simulink model "Neww"  (R2016a)
settings: Solver=VariableStepAuto  StartTime=0.0  StopTime=4  RelTol=1e-3
libraries: fl_lib x10, elec_lib x5, simrfV2util1 x1, nesl_utility x1
settings Model: Creator=syf  LastModifiedBy=syf
settings DebuggingCC: AlgebraicLoopMsg=none  ArtificialAlgebraicLoopMsg=none

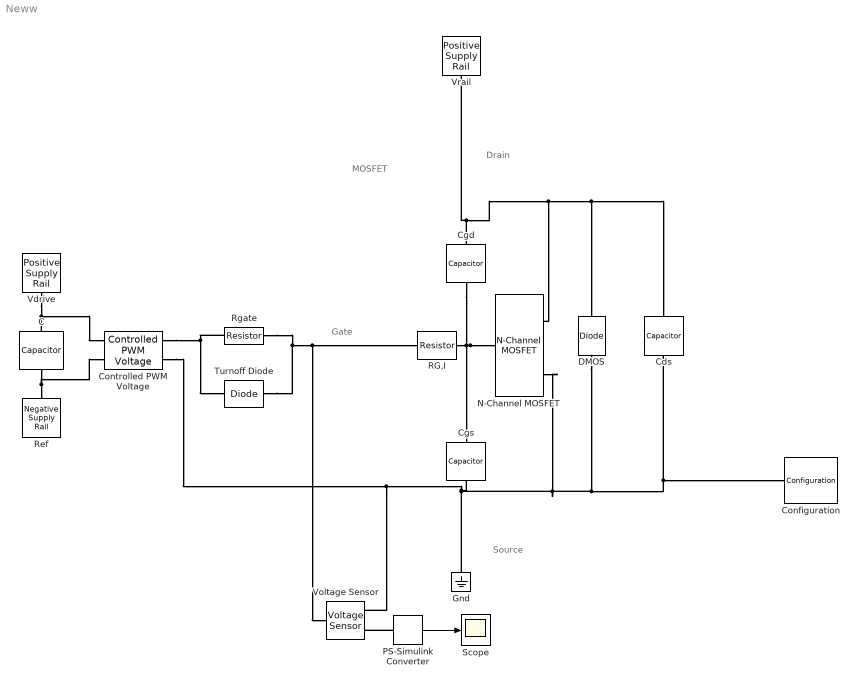
== system Neww ==
  note: Source
  note: Drain
  note: Gate
  note: MOSFET
  C : fl_lib/Electrical/Electrical Elements/Capacitor  c=0.4e-9 F  r=1e-6 Ohm  g=0 1/Ohm  i_specify=off  i_priority=None  i=0 A  v_specify=off  v_priority=None  v=0 V  vc_specify=off  vc_priority=High  vc=0 V
  Cds : fl_lib/Electrical/Electrical Elements/Capacitor  c=0.4e-9 F  r=1e-6 Ohm  g=0 1/Ohm  i_specify=off  i_priority=None  i=0 A  v_specify=off  v_priority=None  v=0 V  vc_specify=off  vc_priority=High  vc=0 V
  Cgd : fl_lib/Electrical/Electrical Elements/Capacitor  c=0.4e-9 F  r=1e-6 Ohm  g=0 1/Ohm  i_specify=off  i_priority=None  i=0 A  v_specify=off  v_priority=None  v=0 V  vc_specify=off  vc_priority=High  vc=0 V
  Cgs : fl_lib/Electrical/Electrical Elements/Capacitor  c=0.4e-9 F  r=1e-6 Ohm  g=0 1/Ohm  i_specify=off  i_priority=None  i=0 A  v_specify=off  v_priority=None  v=0 V  vc_specify=off  vc_priority=High  vc=0 V
  Configuration : simrfV2util1/Configuration  AutoFreq=on  Tones=[] Hz  Harmonics=[]  NormalizeCarrierPower=on  SolverType=Auto  StepSize=1e-6 s  AddNoise=on  Temperature=290.0 K  SolverDelFlag=0
  Controlled PWM Voltage : elec_lib/Actuators & Drivers/Drivers/Controlled PWM Voltage  F=1000 Hz  TD=0 s  pulse_width_offset=0 s  Vmin=0 V  Vmax=5 V  Vm=5 V  pwm_or_av=1  event_type=1  sample_time=1e-6 s
  DMOS : fl_lib/Electrical/Electrical Elements/Diode  Vf=0.6 V  Ron=0.1 Ohm  Goff=1e-8 1/Ohm  i_specify=off  i_priority=None  i=0 A  v_specify=off  v_priority=None  v=0 V
  Gnd : fl_lib/Electrical/Electrical Elements/Electrical Reference
  N-Channel MOSFET : elec_lib/Semiconductor Devices/N-Channel MOSFET  parameterization=1  prmDatasheet=1  prmEquCoeff=1  Beta=5 A/V^2  Rds=0.025 Ohm  Id=6 A  Vgs=10 V  Vth=1.3 V  lam=0 1/V  Tmeas=25 degC  RS=1e-4 Ohm  RD=0.01 Ohm  C_param=1  C_GS=270 pF  C_GD=80 pF  C_DS=0 pF  C_iss=350 pF  C_rss=80 pF  C_oss=0 pF  C_GS_vec=[ 270 300 290 280 295 255 ] pF  C_GD_vec=[ 450 400 300 190 95 55 ] pF  C_DS_vec=[ 450 410 390 230 175 115 ] pF  C_iss_vec=[ 720 700 590 470 390 310 ] pF  C_rss_vec=[ 450 400 300 190 95 55 ] pF  C_oss_vec=[ 900 810 690 420 270 170 ] pF  C_Vds_vec=[ 0.1 0.3 1 3 10 30 ] V  charge_linearity_param=1  C_OX=200 pF  V_C_OX=-0.5 V  dVth_dT=-6 mV/K  Rds_T2=0.037 Ohm  Tmeas2=125 degC  BEXDatasheet=-1.5  BEXEquCoeff=-1.5  TdeviceDatasheet=25 degC  TdeviceEquCoeff=25 degC  Rth=[ 0 10 ] K/W  thermal_mass_parameterization=1  thermal_mass=[ 0 1 ] J/K  thermal_time_constant=[ 0 10 ] s  thermal_mass_initial_temperatures=[ 25 25 ] degC
  PS-Simulink Converter : nesl_utility/PS-Simulink Converter  PhysicalDomain=network_engine_domain  SubClassName=ps_output  LeftPortType=input  RightPortType=output  PseudoPeriodic=off  Frequencies=[]  Unit=1  AffineConversion=off
  RG,I : fl_lib/Electrical/Electrical Elements/Resistor  R=1.5 Ohm  i_specify=off  i_priority=None  i=0 A  v_specify=off  v_priority=None  v=0 V
  Ref : elec_lib/Sources/Negative Supply Rail  v0=0 V
  Rgate : fl_lib/Electrical/Electrical Elements/Resistor  R=1 Ohm  i_specify=off  i_priority=None  i=0 A  v_specify=off  v_priority=None  v=0 V
  Scope : Scope
  Turnoff Diode : fl_lib/Electrical/Electrical Elements/Diode  Vf=0.6 V  Ron=0.1 Ohm  Goff=1e-8 1/Ohm  i_specify=off  i_priority=None  i=0 A  v_specify=off  v_priority=None  v=0 V
  Vdrive : elec_lib/Sources/Positive Supply Rail  v0=10 V
  Voltage Sensor : fl_lib/Electrical/Electrical Sensors/Voltage Sensor
  Vrail : elec_lib/Sources/Positive Supply Rail  v0=450 V
  wires:
  PS-Simulink Converter/1 -> Scope/1
  connections:
  Rgate/LConn1 -- Controlled PWM Voltage/RConn1 -- Turnoff Diode/RConn1
  Rgate/RConn1 -- Turnoff Diode/LConn1 -- RG,I/LConn1 -- Voltage Sensor/LConn1
  RG,I/RConn1 -- Cgd/RConn1 -- Cgs/LConn1 -- N-Channel MOSFET/LConn1
  DMOS/LConn1 -- Cds/RConn1 -- Configuration/LConn1 -- N-Channel MOSFET/RConn2 -- Voltage Sensor/RConn2 -- Controlled PWM Voltage/RConn2 -- Cgs/RConn1 -- Gnd/LConn1
  Cgd/LConn1 -- Vrail/RConn1 -- Cds/LConn1 -- DMOS/RConn1 -- N-Channel MOSFET/RConn1
  C/LConn1 -- Vdrive/RConn1 -- Controlled PWM Voltage/LConn1
  C/RConn1 -- Controlled PWM Voltage/LConn2 -- Ref/LConn1
  PS-Simulink Converter/LConn1 -- Voltage Sensor/RConn1
